simulink model "testing"  (R2023a)
settings: Solver=FixedStepAuto  StartTime=0.0  StopTime=5  FixedStep=0.00025  RelTol=1e-3
InitFcn:
  | addpath(fullfile(matlabroot,'toolbox/physmod/sm/sli/m'))
model workspace (MAT data in the model file):
  battery_cap = 500
  load = 500
libraries: fl_lib x73, ee_lib x11, nesl_utility x6, batteryecm_lib x2
settings Model: Creator=mluser  LastModifiedBy=mluser
settings OptimizationCC: ReuseModelBlockBuffer=off
settings SimscapeCC: SimscapeLogType=all  SimscapeLogLimitData=off

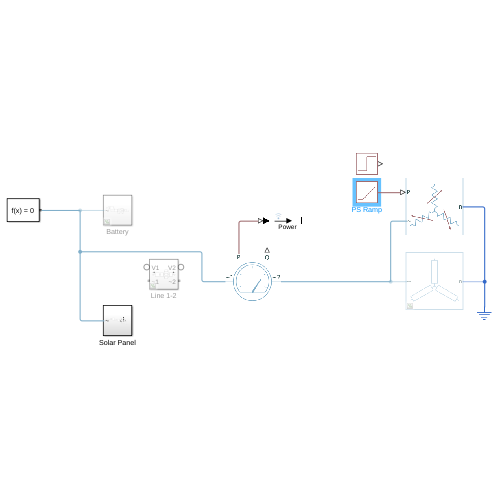
[thumbnail: Simulink's stored preview of the top-level diagram]
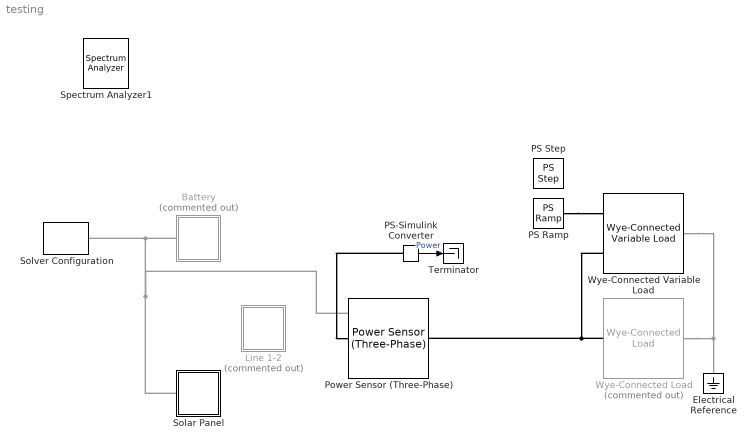
== system testing ==
  Battery : Subsystem  Commented=on
  Electrical Reference : fl_lib/Electrical/Electrical Elements/Electrical Reference
  Line 1-2 : Subsystem  Commented=on
  PS Ramp : fl_lib/Physical Signals/Sources/PS Ramp  slope=200 MW/s  start_time=0 s  initial_output=0 MW
  PS Step : fl_lib/Physical Signals/Sources/PS Step  step_time=1 s  initial_value=400 MW  final_value=1000 MW
  PS-Simulink Converter : nesl_utility/PS-Simulink Converter  PhysicalDomain=network_engine_domain  SubClassName=ps_output  LeftPortType=input  RightPortType=output  PseudoPeriodic=off  Frequencies=[]  VectorFormat=inherit  Unit=inherit  AffineConversion=off
  Power Sensor (Three-Phase) : ee_lib/Sensors & Transducers/Power Sensor (Three-Phase)  load_type=ee.enum.passive.type_balanced.balanced  f0=60 Hz  config=ee.enum.with_neutral.no  rho=1
      settings: InternalSimscapePortConfiguration="{\"Bottom\":[],\"Left\":[{\"id\":\"N1\",\"label\":\"~1\",\"type\":\"foundation.electrical.three_phase\"}],\"Right\":[{\"id\":\"N2\",\"label\":\"~2\",\"type\":\"foundation.electrical.three_phase\"}],\"Top\":[{\"id\":\"Pm\",\"label\":\"P\",\"type\":\"output\"},{\"id\":\"Qm\",\"label\":\"Q\",\"type\":\"output\"}]}"
  Solar Panel : Subsystem
  Solver Configuration : nesl_utility/Solver Configuration  PhysicalDomain=network_engine_domain  SubClassName=solver  LeftPortType=input  RightPortType=generic  Tones=[]  Harmonics=[]  SimulateNoise=off  Profile=off  UseLocalSampling=off  EnableSwitchedLinearOptims=on  FrequencyDomain=off  UseCCode=off  RelTol=0.001  AbsTol=0.001  MinStep=1e-09  ToWorkspace=off  RevertToSquareIcSolve=off  NumHomotopyIterations=100  PhasorMode=off  PhasorModeNumHarmonics=1  ConsistencySolver=NEWTON_XTOL_AFTER_FTOL  IndexReductionMethod=DerivativeReplacement  DoDC=off  ResidualTolerance=1e-09  ConsistencyTolSource=GLOBAL  ConsistencyAbsTol=0.001  ConsistencyRelTol=0.001  ConsistencyTolFactor=0.001  UseLocalSolver=off  LocalSolverChoice=NE_BACKWARD_EULER_ADVANCER  ResolveIndetEquations=on  FunctionEvalNumThread=1  LocalSolverSampleTime=0.001  DoFixedCost=off  MaxNonlinIter=3  MaxModeIter=2  ComputeImpulses=off  ImpulseIterations=2  LinearAlgebra=auto  LinearAlgebraNumThread=0  EquationFormulation=NE_TIME_EF  DelaysMemoryBudget=1024  AutomaticFiltering=on  FilteringTimeConstant=0.001  PartitionStorageMethod=AS_NEEDED  PartitionMemoryBudget=1024  PartitionMethod=ROBUST
  Terminator : Terminator
  Wye-Connected Variable Load : ee_lib/Passive/RLC Assemblies/Wye-Connected Variable Load  VRated=350*sqrt(3) kV  Pmin=1000 W
      settings: InternalSimscapePortConfiguration="{\"Bottom\":[],\"Left\":[{\"id\":\"P\",\"label\":\"P\",\"type\":\"input\"},{\"id\":\"N\",\"label\":\"~\",\"type\":\"foundation.electrical.three_phase\"}],\"Right\":[{\"id\":\"n\",\"label\":\"n\",\"type\":\"foundation.electrical.electrical\"}],\"Top\":[]}"
  Wye-Connected Load : ee_lib/Passive/RLC Assemblies/Wye-Connected Load  Commented=on  parameterization=ee.enum.rlc.parameterization.ratedpower  component_structure=ee.enum.rlc.structure.R  component_structure_PQ=ee.enum.rlc.structure.R  R=1 Ohm  L=1e-3 H  C=1e-6 F  VRated=350*sqrt(3) kV  FRated=60 Hz  P=load MW  Qpos=1e2 A*V  Qneg=-1e2 A*V  R_parasitic=0 Ohm  G_parasitic=0 1/Ohm  R_parasitic_PQ=0 Ohm  G_parasitic_PQ=0 1/Ohm  Vmag0=24e3 V  Vang0=0 deg  Freq0=60 Hz  IL_specify=off  IL_priority=High  IL=[0, 0, 0] A  IL_nominal_specify=off  IL_nominal_unit=A  IL_nominal_value=1  VC_specify=off  VC_priority=High  VC=[0, 0, 0] V  VC_nominal_specify=off  VC_nominal_unit=V  VC_nominal_value=1
  Spectrum Analyzer1 : SpectrumAnalyzer  IOType=viewer  WindowPosition=[692 368 558 418]  Method=Welch  AveragingMethod=Running
      settings: OpenAtSimulationStart=off
  wires:
  PS-Simulink Converter/1 -> Terminator/1  "Power"
  connections:
  Battery/LConn1 -- Power Sensor (Three-Phase)/LConn1 -- Solar Panel/LConn1 -- Solver Configuration/RConn1
  Wye-Connected Variable Load/LConn2 -- Power Sensor (Three-Phase)/RConn1 -- Wye-Connected Load/LConn1
  PS Ramp/RConn1 -- Wye-Connected Variable Load/LConn1
  Wye-Connected Load/RConn1 -- Electrical Reference/LConn1 -- Wye-Connected Variable Load/RConn1
  PS-Simulink Converter/LConn1 -- Power Sensor (Three-Phase)/LConn2

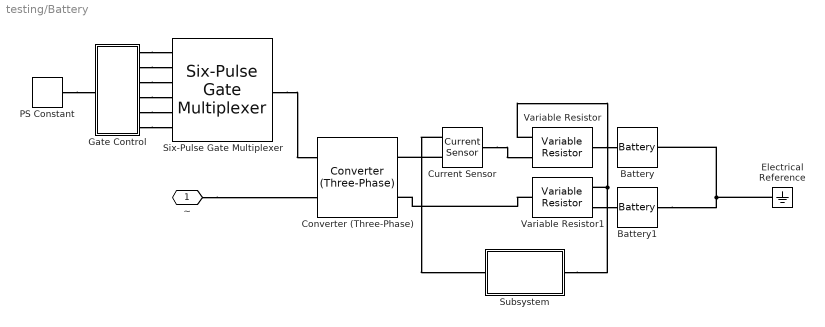
== system testing/Battery ==
  Battery : batteryecm_lib/Battery  Vnom=494.97 kV  prm_dir=simscape.enum.battery.prm_dir.disabled  R1_dis=2 Ohm  R1_ch=2 Ohm  R1=0.17 Ohm  prm_AH=simscape.enum.battery.prm_AH.infinite  AH=50 A*hr  V1=11.5 V  AH1=25 A*hr  prm_R2=simscape.enum.battery.prm_R2.disabled  R2=2000 Ohm  Tmeas=298.15 K  charge_measurement_port=simscape.enum.battery.enable.no  prm_dyn=simscape.enum.battery.prm_dyn.off  Rp1=0.005 Ohm  tau1=30 s  Rp2=0.005 Ohm  tau2=30 s  Rp3=0.005 Ohm  tau3=30 s  Rp4=0.005 Ohm  tau4=30 s  Rp5=0.005 Ohm  tau5=30 s  prm_fade=simscape.enum.battery.prm_fade.disabled  N_fade=100  AH_fade=45 A*hr  R1_fade=2.02 Ohm  R1_ch_fade=2.02 Ohm  V1_fade=10.35 V  prm_age=simscape.enum.battery.prm_age.disabled  prm_age_OCV=simscape.enum.battery.prm_age_OCV.OCV  OCV_age=0.9  SOC_age=60  Tmeas_age=298.15 K  delta_time_age_vec=[0] d  temperature_age_vec=[273] K  OCV_scaling_age=2.2134e6  OCV_offset_age=1.632e6  temp_exp_age=0.515833569 V  t_exp_age=0.75  Vnom_T2=12 V  R1_T2=2.2 Ohm  R1_T2_dis=2.2 Ohm  R1_T2_ch=2.2 Ohm  V1_T2=11.4 V  R2_T2=2200 Ohm  Rp1_T2=0.005 Ohm  tau1_T2=30 s  Rp2_T2=0.005 Ohm  tau2_T2=30 s  Rp3_T2=0.005 Ohm  tau3_T2=30 s  Rp4_T2=0.005 Ohm  tau4_T2=30 s  Rp5_T2=0.005 Ohm  tau5_T2=30 s  Tmeas2=273.15 K  thermal_port=simscape.enum.thermaleffects.omit  thermal_mass=30000 J/K  i_specify=off  i_priority=None  i=0 A  i_nominal_specify=off  i_nominal_unit=A  i_nominal_value=1  v_specify=off  v_priority=None  v=0 V  v_nominal_specify=off  v_nominal_unit=V  v_nominal_value=1  charge_specify=off  charge_priority=High  charge=50 A*hr  charge_nominal_specify=off  charge_nominal_unit=A*hr  charge_nominal_value=1  num_cycles_specify=off  num_cycles_priority=High  num_cycles=0  num_cycles_nominal_specify=off  num_cycles_nominal_unit=1  num_cycles_nominal_value=1  temperature_specify=off  temperature_priority=High  temperature=298.15 K  temperature_nominal_specify=off  temperature_nominal_unit=K  temperature_nominal_value=1
  Battery1 : batteryecm_lib/Battery  Vnom=494.97 kV  prm_dir=simscape.enum.battery.prm_dir.disabled  R1_dis=2 Ohm  R1_ch=2 Ohm  R1=0.17 Ohm  prm_AH=simscape.enum.battery.prm_AH.infinite  AH=50 A*hr  V1=11.5 V  AH1=25 A*hr  prm_R2=simscape.enum.battery.prm_R2.disabled  R2=2000 Ohm  Tmeas=298.15 K  charge_measurement_port=simscape.enum.battery.enable.no  prm_dyn=simscape.enum.battery.prm_dyn.off  Rp1=0.005 Ohm  tau1=30 s  Rp2=0.005 Ohm  tau2=30 s  Rp3=0.005 Ohm  tau3=30 s  Rp4=0.005 Ohm  tau4=30 s  Rp5=0.005 Ohm  tau5=30 s  prm_fade=simscape.enum.battery.prm_fade.disabled  N_fade=100  AH_fade=45 A*hr  R1_fade=2.02 Ohm  R1_ch_fade=2.02 Ohm  V1_fade=10.35 V  prm_age=simscape.enum.battery.prm_age.disabled  prm_age_OCV=simscape.enum.battery.prm_age_OCV.OCV  OCV_age=0.9  SOC_age=60  Tmeas_age=298.15 K  delta_time_age_vec=[0] d  temperature_age_vec=[273] K  OCV_scaling_age=2.2134e6  OCV_offset_age=1.632e6  temp_exp_age=0.515833569 V  t_exp_age=0.75  Vnom_T2=12 V  R1_T2=2.2 Ohm  R1_T2_dis=2.2 Ohm  R1_T2_ch=2.2 Ohm  V1_T2=11.4 V  R2_T2=2200 Ohm  Rp1_T2=0.005 Ohm  tau1_T2=30 s  Rp2_T2=0.005 Ohm  tau2_T2=30 s  Rp3_T2=0.005 Ohm  tau3_T2=30 s  Rp4_T2=0.005 Ohm  tau4_T2=30 s  Rp5_T2=0.005 Ohm  tau5_T2=30 s  Tmeas2=273.15 K  thermal_port=simscape.enum.thermaleffects.omit  thermal_mass=30000 J/K  i_specify=off  i_priority=None  i=0 A  i_nominal_specify=off  i_nominal_unit=A  i_nominal_value=1  v_specify=off  v_priority=None  v=0 V  v_nominal_specify=off  v_nominal_unit=V  v_nominal_value=1  charge_specify=off  charge_priority=High  charge=50 A*hr  charge_nominal_specify=off  charge_nominal_unit=A*hr  charge_nominal_value=1  num_cycles_specify=off  num_cycles_priority=High  num_cycles=0  num_cycles_nominal_specify=off  num_cycles_nominal_unit=1  num_cycles_nominal_value=1  temperature_specify=off  temperature_priority=High  temperature=298.15 K  temperature_nominal_specify=off  temperature_nominal_unit=K  temperature_nominal_value=1
  Converter (Three-Phase) : ee_lib/Semiconductors & Converters/Converters/Converter (Three-Phase)  port_option=ee.enum.threePhasePort.composite  device_type=ee.enum.converters.switchingdevice.averaged  K=0  Vf=0.8 V  Ron=1e-9 mOhm  Rds=0.001 Ohm  Goff=1e-6 1/Ohm  Vgt=1 V  Vgt_off=-1 V  Ih=1 A  Vth=6 V  diode_param=ee.enum.converters.protectiondiode.none  diode_Vf=1 MV  diode_Ron=0.001 Ohm  diode_Goff=1e-5 1/Ohm  diode_C=50 nF  diode_iRM=-235 A  diode_iF=300 A  diode_idot=-50 A/us  diode_trr_param=ee.enum.converters.diodetrr.trr_factor  diode_trr_factor=3  diode_trr=15 us  diode_Qrr=1500 s*uA  snubber_type=ee.enum.converters.snubber.exclude  Cs=1e-7 F  Rs=0.1 Ohm
  Current Sensor : fl_lib/Electrical/Electrical Sensors/Current Sensor
  Electrical Reference : fl_lib/Electrical/Electrical Elements/Electrical Reference
  Gate Control : Subsystem
  PS Constant : fl_lib/Physical Signals/Sources/PS Constant  constant=1
  Six-Pulse Gate Multiplexer : ee_lib/Semiconductors & Converters/Converters/Six-Pulse Gate Multiplexer  port_option=ee.enum.controlport.ps
  Subsystem : Subsystem
  Variable Resistor : fl_lib/Electrical/Electrical Elements/Variable Resistor  Rmin=0 Ohm  i_specify=off  i_priority=None  i=0 A  i_nominal_specify=off  i_nominal_unit=A  i_nominal_value=1  v_specify=off  v_priority=None  v=0 V  v_nominal_specify=off  v_nominal_unit=V  v_nominal_value=1
  Variable Resistor1 : fl_lib/Electrical/Electrical Elements/Variable Resistor  Rmin=0 Ohm  i_specify=off  i_priority=None  i=0 A  i_nominal_specify=off  i_nominal_unit=A  i_nominal_value=1  v_specify=off  v_priority=None  v=0 V  v_nominal_specify=off  v_nominal_unit=V  v_nominal_value=1
  ~ : PMIOPort  Side=Left
  connections:
  Six-Pulse Gate Multiplexer/RConn1 -- Converter (Three-Phase)/LConn1
  ~/RConn1 -- Converter (Three-Phase)/LConn2
  Gate Control/RConn1 -- Six-Pulse Gate Multiplexer/LConn1
  Gate Control/RConn2 -- Six-Pulse Gate Multiplexer/LConn2
  Gate Control/RConn3 -- Six-Pulse Gate Multiplexer/LConn3
  Gate Control/RConn4 -- Six-Pulse Gate Multiplexer/LConn4
  Gate Control/RConn5 -- Six-Pulse Gate Multiplexer/LConn5
  Gate Control/RConn6 -- Six-Pulse Gate Multiplexer/LConn6
  PS Constant/RConn1 -- Gate Control/LConn1
  Battery1/LConn1 -- Battery/RConn1 -- Electrical Reference/LConn1
  Current Sensor/RConn2 -- Converter (Three-Phase)/RConn1
  Variable Resistor/RConn1 -- Battery/LConn1
  Variable Resistor1/RConn1 -- Converter (Three-Phase)/RConn2
  Variable Resistor1/LConn2 -- Battery1/RConn1
  Current Sensor/LConn1 -- Variable Resistor/LConn2
  Current Sensor/RConn1 -- Subsystem/LConn1
  Subsystem/RConn1 -- Variable Resistor/LConn1 -- Variable Resistor1/LConn1

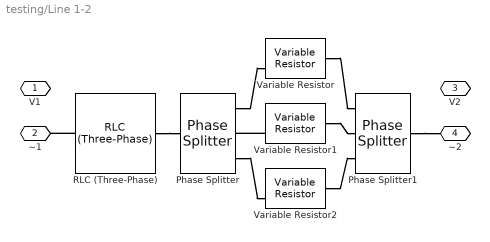
== system testing/Line 1-2 ==
  Phase Splitter : ee_lib/Connectors & References/Phase Splitter
  Phase Splitter1 : ee_lib/Connectors & References/Phase Splitter
  RLC (Three-Phase) : ee_lib/Passive/RLC Assemblies/RLC (Three-Phase)  component_structure=ee.enum.rlc.structure.SeriesRL  R=10 Ohm  L=5e-3 H  C=1e-6 F  R_parasitic=0 Ohm  G_parasitic=0 1/Ohm  IL_specify=off  IL_priority=High  IL=[0, 0, 0] A  IL_nominal_specify=off  IL_nominal_unit=A  IL_nominal_value=1  VC_specify=off  VC_priority=High  VC=[0, 0, 0] V  VC_nominal_specify=off  VC_nominal_unit=V  VC_nominal_value=1
      settings: InternalSimscapePortConfiguration="{\"Bottom\":[],\"Left\":[{\"id\":\"N1\",\"label\":\"~1\",\"type\":\"foundation.electrical.three_phase\"}],\"Right\":[{\"id\":\"N2\",\"label\":\"~2\",\"type\":\"foundation.electrical.three_phase\"}],\"Top\":[]}"
  Variable Resistor : fl_lib/Electrical/Electrical Elements/Variable Resistor  Rmin=0 Ohm  i_specify=off  i_priority=None  i=0 A  i_nominal_specify=off  i_nominal_unit=A  i_nominal_value=1  v_specify=off  v_priority=None  v=0 V  v_nominal_specify=off  v_nominal_unit=V  v_nominal_value=1
  Variable Resistor1 : fl_lib/Electrical/Electrical Elements/Variable Resistor  Rmin=0 Ohm  i_specify=off  i_priority=None  i=0 A  i_nominal_specify=off  i_nominal_unit=A  i_nominal_value=1  v_specify=off  v_priority=None  v=0 V  v_nominal_specify=off  v_nominal_unit=V  v_nominal_value=1
  Variable Resistor2 : fl_lib/Electrical/Electrical Elements/Variable Resistor  Rmin=0 Ohm  i_specify=off  i_priority=None  i=0 A  i_nominal_specify=off  i_nominal_unit=A  i_nominal_value=1  v_specify=off  v_priority=None  v=0 V  v_nominal_specify=off  v_nominal_unit=V  v_nominal_value=1
  V1 : PMIOPort  Side=Left
  ~1 : PMIOPort  Port=2  Side=Left
  V2 : PMIOPort  Port=3  Side=Right
  ~2 : PMIOPort  Port=4  Side=Right
  connections:
  RLC (Three-Phase)/RConn1 -- Phase Splitter/LConn1
  RLC (Three-Phase)/LConn1 -- ~1/RConn1
  Phase Splitter1/LConn1 -- ~2/RConn1
  Phase Splitter/RConn1 -- Variable Resistor/LConn2
  Variable Resistor/RConn1 -- Phase Splitter1/RConn1
  Variable Resistor1/LConn2 -- Phase Splitter/RConn2
  Variable Resistor1/RConn1 -- Phase Splitter1/RConn2
  Phase Splitter/RConn3 -- Variable Resistor2/LConn2
  Variable Resistor2/RConn1 -- Phase Splitter1/RConn3

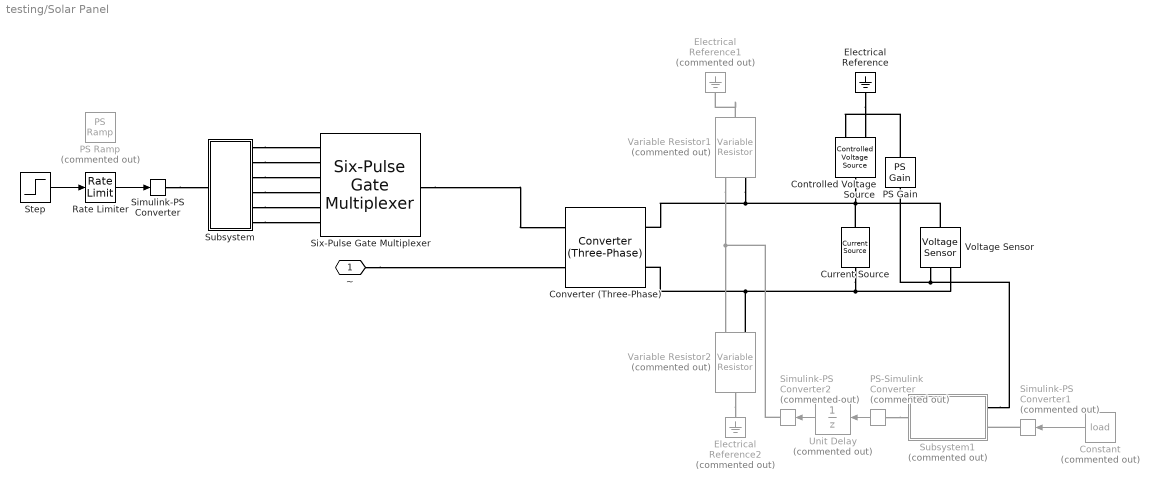
== system testing/Solar Panel ==
  Constant : Constant  Commented=on  Value=load  VectorParams1D=off
  Controlled Voltage Source : fl_lib/Electrical/Electrical Sources/Controlled Voltage Source
  Converter (Three-Phase) : ee_lib/Semiconductors & Converters/Converters/Converter (Three-Phase)  port_option=ee.enum.threePhasePort.composite  device_type=ee.enum.converters.switchingdevice.averaged  K=0  Vf=0.8 V  Ron=1e-9 Ohm  Rds=0.001 Ohm  Goff=1e-6 1/Ohm  Vgt=1 V  Vgt_off=-1 V  Ih=1 A  Vth=6 V  diode_param=ee.enum.converters.protectiondiode.none  diode_Vf=1 MV  diode_Ron=0.001 Ohm  diode_Goff=1e-5 1/Ohm  diode_C=50 nF  diode_iRM=-235 A  diode_iF=300 A  diode_idot=-50 A/us  diode_trr_param=ee.enum.converters.diodetrr.trr_factor  diode_trr_factor=3  diode_trr=15 us  diode_Qrr=1500 s*uA  snubber_type=ee.enum.converters.snubber.exclude  Cs=1e-7 F  Rs=0.1 Ohm
  Current Source : ee_lib/Sources/Current Source  dc_current=load/(2*350*sqrt(2)) kA  ac_current=0 A  ac_shift=0 rad  ac_frequency=60 Hz  noise_mode=ee.enum.sources.noise.Disabled  PSD=0 A^2/Hz  sample_time=1e-3 s  repeatability=ee.enum.sources.repeatability.NotRepeatable  user_seed=0  auto_seed=2715962282  i_specify=off  i_priority=None  i=0 A  i_nominal_specify=off  i_nominal_unit=A  i_nominal_value=1  v_specify=off  v_priority=None  v=0 V  v_nominal_specify=off  v_nominal_unit=V  v_nominal_value=1
  Electrical Reference : fl_lib/Electrical/Electrical Elements/Electrical Reference
  Electrical Reference1 : fl_lib/Electrical/Electrical Elements/Electrical Reference  Commented=on
  Electrical Reference2 : fl_lib/Electrical/Electrical Elements/Electrical Reference  Commented=on
  PS Gain : fl_lib/Physical Signals/Functions/PS Gain  gain=0.5
  PS Ramp : fl_lib/Physical Signals/Sources/PS Ramp  Commented=on  slope=0.1 1/s  start_time=1 s  initial_output=1
  PS-Simulink Converter : nesl_utility/PS-Simulink Converter  Commented=on  PhysicalDomain=network_engine_domain  SubClassName=ps_output  LeftPortType=input  RightPortType=output  PseudoPeriodic=off  Frequencies=[]  VectorFormat=inherit  Unit=inherit  AffineConversion=off
  Rate Limiter : RateLimiter  RisingSlewLimit=0.3  FallingSlewLimit=-0.3  SampleTimeMode=inherited
  Simulink-PS Converter : nesl_utility/Simulink-PS Converter  PhysicalDomain=network_engine_domain  SubClassName=ps_input  LeftPortType=input  RightPortType=output  PseudoPeriodic=off  Frequencies=[]  NoiseDistribution=none  NoiseParameters=[]  Unit=1  AffineConversion=off  FilteringAndDerivatives=provide  SimscapeFilterOrder=1  InputFilterTimeConstant=0.001  UdotUserProvided=0
  Simulink-PS Converter1 : nesl_utility/Simulink-PS Converter  Commented=on  PhysicalDomain=network_engine_domain  SubClassName=ps_input  LeftPortType=input  RightPortType=output  PseudoPeriodic=off  Frequencies=[]  NoiseDistribution=none  NoiseParameters=[]  Unit=MW  AffineConversion=off  FilteringAndDerivatives=provide  SimscapeFilterOrder=1  InputFilterTimeConstant=0.001  UdotUserProvided=0
  Simulink-PS Converter2 : nesl_utility/Simulink-PS Converter  Commented=on  PhysicalDomain=network_engine_domain  SubClassName=ps_input  LeftPortType=input  RightPortType=output  PseudoPeriodic=off  Frequencies=[]  NoiseDistribution=none  NoiseParameters=[]  Unit=Ohm  AffineConversion=off  FilteringAndDerivatives=provide  SimscapeFilterOrder=1  InputFilterTimeConstant=0.001  UdotUserProvided=0
  Six-Pulse Gate Multiplexer : ee_lib/Semiconductors & Converters/Converters/Six-Pulse Gate Multiplexer  port_option=ee.enum.controlport.ps
  Step : Step  Time=0  Before=1  SampleTime=0
  Subsystem : Subsystem
  Subsystem1 : Subsystem  Commented=on
  Unit Delay : UnitDelay  Commented=on  InitialCondition=1e9  SampleTime=-1  HasFrameUpgradeWarning=on
  Variable Resistor1 : fl_lib/Electrical/Electrical Elements/Variable Resistor  Commented=on  Rmin=0 Ohm  i_specify=off  i_priority=None  i=0 A  i_nominal_specify=off  i_nominal_unit=A  i_nominal_value=1  v_specify=off  v_priority=None  v=0 V  v_nominal_specify=off  v_nominal_unit=V  v_nominal_value=1
  Variable Resistor2 : fl_lib/Electrical/Electrical Elements/Variable Resistor  Commented=on  Rmin=0 Ohm  i_specify=off  i_priority=None  i=0 A  i_nominal_specify=off  i_nominal_unit=A  i_nominal_value=1  v_specify=off  v_priority=None  v=0 V  v_nominal_specify=off  v_nominal_unit=V  v_nominal_value=1
  Voltage Sensor : fl_lib/Electrical/Electrical Sensors/Voltage Sensor
  ~ : PMIOPort  Side=Left
  wires:
  Rate Limiter/1 -> Simulink-PS Converter/1
  Step/1 -> Rate Limiter/1
  Constant/1 -> Simulink-PS Converter1/1
  PS-Simulink Converter/1 -> Unit Delay/1
  Unit Delay/1 -> Simulink-PS Converter2/1
  connections:
  Voltage Sensor/RConn2 -- Current Source/RConn1 -- Variable Resistor2/LConn2 -- Converter (Three-Phase)/RConn2
  Voltage Sensor/LConn1 -- Current Source/LConn1 -- Converter (Three-Phase)/RConn1 -- Variable Resistor1/LConn2 -- Controlled Voltage Source/LConn1
  Voltage Sensor/RConn1 -- Subsystem1/LConn1 -- PS Gain/LConn1
  ~/RConn1 -- Converter (Three-Phase)/LConn2
  Six-Pulse Gate Multiplexer/RConn1 -- Converter (Three-Phase)/LConn1
  PS Gain/RConn1 -- Controlled Voltage Source/RConn1
  Electrical Reference/LConn1 -- Controlled Voltage Source/RConn2
  Subsystem/RConn1 -- Six-Pulse Gate Multiplexer/LConn1
  Subsystem/RConn2 -- Six-Pulse Gate Multiplexer/LConn2
  Subsystem/RConn3 -- Six-Pulse Gate Multiplexer/LConn3
  Subsystem/RConn4 -- Six-Pulse Gate Multiplexer/LConn4
  Subsystem/RConn5 -- Six-Pulse Gate Multiplexer/LConn5
  Subsystem/RConn6 -- Six-Pulse Gate Multiplexer/LConn6
  Simulink-PS Converter/RConn1 -- Subsystem/LConn1
  Variable Resistor1/RConn1 -- Electrical Reference1/LConn1
  Variable Resistor2/RConn1 -- Electrical Reference2/LConn1
  Simulink-PS Converter1/RConn1 -- Subsystem1/LConn2
  PS-Simulink Converter/LConn1 -- Subsystem1/RConn1
  Simulink-PS Converter2/RConn1 -- Variable Resistor2/LConn1 -- Variable Resistor1/LConn1

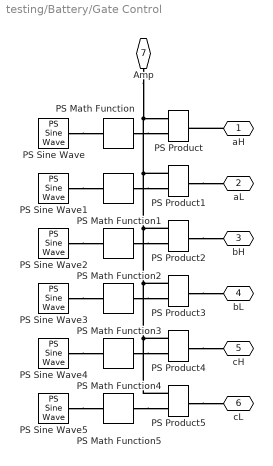
== system testing/Battery/Gate Control ==
  PS Math Function{,1..5} (6 alike) : fl_lib/Physical Signals/Functions/PS Math Function  fcn_choice=foundation.enum.math_function.square  v=1
  PS Product{,1..5} (6 alike) : fl_lib/Physical Signals/Functions/PS Product
  PS Sine Wave : fl_lib/Physical Signals/Sources/PS Sine Wave  amplitude=1  bias=0  frequency_spec=foundation.enum.frequencySpec.frequencySI  frequency_SI=30 Hz  frequency_angular=1 rad/s  phase=pi/2 rad
      settings: InternalSimscapePortConfiguration="{\"Bottom\":[],\"Left\":[],\"Right\":[{\"id\":\"O\",\"label\":\"\",\"type\":\"output\"}],\"Top\":[]}"
  PS Sine Wave1 : fl_lib/Physical Signals/Sources/PS Sine Wave  amplitude=1  bias=0  frequency_spec=foundation.enum.frequencySpec.frequencySI  frequency_SI=30 Hz  frequency_angular=1 rad/s  phase=0 rad
      settings: InternalSimscapePortConfiguration="{\"Bottom\":[],\"Left\":[],\"Right\":[{\"id\":\"O\",\"label\":\"\",\"type\":\"output\"}],\"Top\":[]}"
  PS Sine Wave2 : fl_lib/Physical Signals/Sources/PS Sine Wave  amplitude=1  bias=0  frequency_spec=foundation.enum.frequencySpec.frequencySI  frequency_SI=30 Hz  frequency_angular=1 rad/s  phase=2*pi/3+pi/2 rad
      settings: InternalSimscapePortConfiguration="{\"Bottom\":[],\"Left\":[],\"Right\":[{\"id\":\"O\",\"label\":\"\",\"type\":\"output\"}],\"Top\":[]}"
  PS Sine Wave3 : fl_lib/Physical Signals/Sources/PS Sine Wave  amplitude=1  bias=0  frequency_spec=foundation.enum.frequencySpec.frequencySI  frequency_SI=30 Hz  frequency_angular=1 rad/s  phase=2*pi/3 rad
      settings: InternalSimscapePortConfiguration="{\"Bottom\":[],\"Left\":[],\"Right\":[{\"id\":\"O\",\"label\":\"\",\"type\":\"output\"}],\"Top\":[]}"
  PS Sine Wave4 : fl_lib/Physical Signals/Sources/PS Sine Wave  amplitude=1  bias=0  frequency_spec=foundation.enum.frequencySpec.frequencySI  frequency_SI=30 Hz  frequency_angular=1 rad/s  phase=-2*pi/3+pi/2 rad
      settings: InternalSimscapePortConfiguration="{\"Bottom\":[],\"Left\":[],\"Right\":[{\"id\":\"O\",\"label\":\"\",\"type\":\"output\"}],\"Top\":[]}"
  PS Sine Wave5 : fl_lib/Physical Signals/Sources/PS Sine Wave  amplitude=1  bias=0  frequency_spec=foundation.enum.frequencySpec.frequencySI  frequency_SI=30 Hz  frequency_angular=1 rad/s  phase=-2*pi/3 rad
      settings: InternalSimscapePortConfiguration="{\"Bottom\":[],\"Left\":[],\"Right\":[{\"id\":\"O\",\"label\":\"\",\"type\":\"output\"}],\"Top\":[]}"
  aH : PMIOPort  Side=Right
  aL : PMIOPort  Port=2  Side=Right
  bH : PMIOPort  Port=3  Side=Right
  bL : PMIOPort  Port=4  Side=Right
  cH : PMIOPort  Port=5  Side=Right
  cL : PMIOPort  Port=6  Side=Right
  Amp : PMIOPort  Port=7  Side=Left
  connections:
  aH/RConn1 -- PS Product/RConn1
  PS Math Function/RConn1 -- PS Product/LConn2
  Amp/RConn1 -- PS Product/LConn1 -- PS Product1/LConn1 -- PS Product2/LConn1 -- PS Product3/LConn1 -- PS Product5/LConn1 -- PS Product4/LConn1
  PS Sine Wave/RConn1 -- PS Math Function/LConn1
  PS Math Function1/RConn1 -- PS Product1/LConn2
  PS Sine Wave1/RConn1 -- PS Math Function1/LConn1
  PS Product1/RConn1 -- aL/RConn1
  PS Math Function2/RConn1 -- PS Product2/LConn2
  PS Sine Wave2/RConn1 -- PS Math Function2/LConn1
  PS Product2/RConn1 -- bH/RConn1
  PS Math Function3/RConn1 -- PS Product3/LConn2
  PS Sine Wave3/RConn1 -- PS Math Function3/LConn1
  PS Product3/RConn1 -- bL/RConn1
  PS Math Function4/RConn1 -- PS Product4/LConn2
  PS Sine Wave4/RConn1 -- PS Math Function4/LConn1
  PS Math Function5/RConn1 -- PS Product5/LConn2
  PS Sine Wave5/RConn1 -- PS Math Function5/LConn1
  PS Product4/RConn1 -- cH/RConn1
  PS Product5/RConn1 -- cL/RConn1

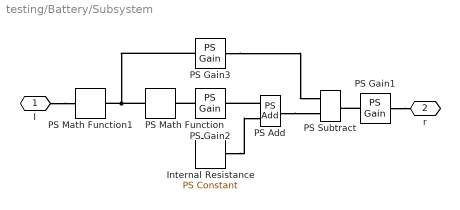
== system testing/Battery/Subsystem ==
  Internal Resistance : fl_lib/Physical Signals/Sources/PS Constant  constant=0.34 Ohm
  PS Add : fl_lib/Physical Signals/Functions/PS Add
  PS Gain1 : fl_lib/Physical Signals/Functions/PS Gain  gain=0.5
  PS Gain2 : fl_lib/Physical Signals/Functions/PS Gain  gain=battery_cap MW
  PS Gain3 : fl_lib/Physical Signals/Functions/PS Gain  gain=2*350*sqrt(2) kV
  PS Math Function : fl_lib/Physical Signals/Functions/PS Math Function  fcn_choice=foundation.enum.math_function.square  v=1
  PS Math Function1 : fl_lib/Physical Signals/Functions/PS Math Function  fcn_choice=foundation.enum.math_function.reciprocal  v=1
  PS Subtract : fl_lib/Physical Signals/Functions/PS Subtract
  I : PMIOPort  Side=Left
  r : PMIOPort  Port=2  Side=Right
  connections:
  I/RConn1 -- PS Math Function1/LConn1
  PS Gain1/LConn1 -- PS Subtract/RConn1
  PS Gain1/RConn1 -- r/RConn1
  PS Add/RConn1 -- PS Subtract/LConn2
  Internal Resistance/RConn1 -- PS Add/LConn2
  PS Math Function/LConn1 -- PS Gain3/LConn1 -- PS Math Function1/RConn1
  PS Gain2/LConn1 -- PS Math Function/RConn1
  PS Add/LConn1 -- PS Gain2/RConn1
  PS Gain3/RConn1 -- PS Subtract/LConn1

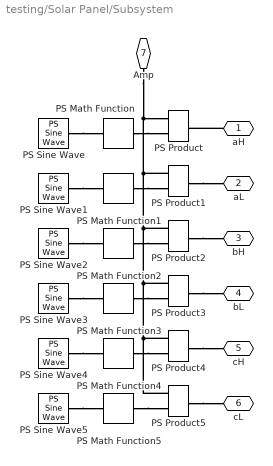
== system testing/Solar Panel/Subsystem ==
  PS Math Function{,1..5} (6 alike) : fl_lib/Physical Signals/Functions/PS Math Function  fcn_choice=foundation.enum.math_function.square  v=1
  PS Product{,1..5} (6 alike) : fl_lib/Physical Signals/Functions/PS Product
  PS Sine Wave : fl_lib/Physical Signals/Sources/PS Sine Wave  amplitude=1  bias=0  frequency_spec=foundation.enum.frequencySpec.frequencySI  frequency_SI=30 Hz  frequency_angular=1 rad/s  phase=pi/2 rad
      settings: InternalSimscapePortConfiguration="{\"Bottom\":[],\"Left\":[],\"Right\":[{\"id\":\"O\",\"label\":\"\",\"type\":\"output\"}],\"Top\":[]}"
  PS Sine Wave1 : fl_lib/Physical Signals/Sources/PS Sine Wave  amplitude=1  bias=0  frequency_spec=foundation.enum.frequencySpec.frequencySI  frequency_SI=30 Hz  frequency_angular=1 rad/s  phase=0 rad
      settings: InternalSimscapePortConfiguration="{\"Bottom\":[],\"Left\":[],\"Right\":[{\"id\":\"O\",\"label\":\"\",\"type\":\"output\"}],\"Top\":[]}"
  PS Sine Wave2 : fl_lib/Physical Signals/Sources/PS Sine Wave  amplitude=1  bias=0  frequency_spec=foundation.enum.frequencySpec.frequencySI  frequency_SI=30 Hz  frequency_angular=1 rad/s  phase=-2*pi/3+pi/2 rad
      settings: InternalSimscapePortConfiguration="{\"Bottom\":[],\"Left\":[],\"Right\":[{\"id\":\"O\",\"label\":\"\",\"type\":\"output\"}],\"Top\":[]}"
  PS Sine Wave3 : fl_lib/Physical Signals/Sources/PS Sine Wave  amplitude=1  bias=0  frequency_spec=foundation.enum.frequencySpec.frequencySI  frequency_SI=30 Hz  frequency_angular=1 rad/s  phase=-2*pi/3 rad
      settings: InternalSimscapePortConfiguration="{\"Bottom\":[],\"Left\":[],\"Right\":[{\"id\":\"O\",\"label\":\"\",\"type\":\"output\"}],\"Top\":[]}"
  PS Sine Wave4 : fl_lib/Physical Signals/Sources/PS Sine Wave  amplitude=1  bias=0  frequency_spec=foundation.enum.frequencySpec.frequencySI  frequency_SI=30 Hz  frequency_angular=1 rad/s  phase=2*pi/3+pi/2 rad
      settings: InternalSimscapePortConfiguration="{\"Bottom\":[],\"Left\":[],\"Right\":[{\"id\":\"O\",\"label\":\"\",\"type\":\"output\"}],\"Top\":[]}"
  PS Sine Wave5 : fl_lib/Physical Signals/Sources/PS Sine Wave  amplitude=1  bias=0  frequency_spec=foundation.enum.frequencySpec.frequencySI  frequency_SI=30 Hz  frequency_angular=1 rad/s  phase=2*pi/3 rad
      settings: InternalSimscapePortConfiguration="{\"Bottom\":[],\"Left\":[],\"Right\":[{\"id\":\"O\",\"label\":\"\",\"type\":\"output\"}],\"Top\":[]}"
  aH : PMIOPort  Side=Right
  aL : PMIOPort  Port=2  Side=Right
  bH : PMIOPort  Port=3  Side=Right
  bL : PMIOPort  Port=4  Side=Right
  cH : PMIOPort  Port=5  Side=Right
  cL : PMIOPort  Port=6  Side=Right
  Amp : PMIOPort  Port=7  Side=Left
  connections:
  aH/RConn1 -- PS Product/RConn1
  PS Math Function/RConn1 -- PS Product/LConn2
  Amp/RConn1 -- PS Product/LConn1 -- PS Product1/LConn1 -- PS Product2/LConn1 -- PS Product3/LConn1 -- PS Product5/LConn1 -- PS Product4/LConn1
  PS Sine Wave/RConn1 -- PS Math Function/LConn1
  PS Math Function1/RConn1 -- PS Product1/LConn2
  PS Sine Wave1/RConn1 -- PS Math Function1/LConn1
  PS Product1/RConn1 -- aL/RConn1
  PS Math Function2/RConn1 -- PS Product2/LConn2
  PS Sine Wave2/RConn1 -- PS Math Function2/LConn1
  PS Product2/RConn1 -- bH/RConn1
  PS Math Function3/RConn1 -- PS Product3/LConn2
  PS Sine Wave3/RConn1 -- PS Math Function3/LConn1
  PS Product3/RConn1 -- bL/RConn1
  PS Math Function4/RConn1 -- PS Product4/LConn2
  PS Sine Wave4/RConn1 -- PS Math Function4/LConn1
  PS Math Function5/RConn1 -- PS Product5/LConn2
  PS Sine Wave5/RConn1 -- PS Math Function5/LConn1
  PS Product4/RConn1 -- cH/RConn1
  PS Product5/RConn1 -- cL/RConn1

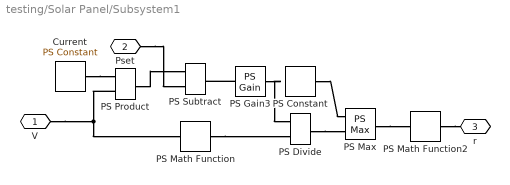
== system testing/Solar Panel/Subsystem1 ==
  Current : fl_lib/Physical Signals/Sources/PS Constant  constant=load/(2*350*sqrt(2)) kA
  PS Constant : fl_lib/Physical Signals/Sources/PS Constant  constant=1e-9 1/Ohm
  PS Divide : fl_lib/Physical Signals/Functions/PS Divide
  PS Gain3 : fl_lib/Physical Signals/Functions/PS Gain  gain=2
  PS Math Function : fl_lib/Physical Signals/Functions/PS Math Function  fcn_choice=foundation.enum.math_function.square  v=1
  PS Math Function2 : fl_lib/Physical Signals/Functions/PS Math Function  fcn_choice=foundation.enum.math_function.reciprocal  v=1
  PS Max : fl_lib/Physical Signals/Nonlinear Operators/PS Max
      settings: InternalSimscapePortConfiguration="{\"Bottom\":[],\"Left\":[{\"id\":\"I1\",\"label\":\"\",\"type\":\"input\"},{\"id\":\"I2\",\"label\":\"\",\"type\":\"input\"}],\"Right\":[{\"id\":\"O\",\"label\":\"\",\"type\":\"output\"}],\"Top\":[]}"
  PS Product : fl_lib/Physical Signals/Functions/PS Product
  PS Subtract : fl_lib/Physical Signals/Functions/PS Subtract
  V : PMIOPort  Side=Left
  Pset : PMIOPort  Port=2  Side=Left
  r : PMIOPort  Port=3  Side=Right
  connections:
  PS Math Function2/RConn1 -- r/RConn1
  V/RConn1 -- PS Product/LConn2 -- PS Math Function/LConn1
  PS Gain3/LConn1 -- PS Subtract/RConn1
  Current/RConn1 -- PS Product/LConn1
  PS Gain3/RConn1 -- PS Divide/LConn1
  PS Math Function/RConn1 -- PS Divide/LConn2
  Pset/RConn1 -- PS Subtract/LConn2
  PS Product/RConn1 -- PS Subtract/LConn1
  PS Max/RConn1 -- PS Math Function2/LConn1
  PS Divide/RConn1 -- PS Max/LConn2
  PS Constant/RConn1 -- PS Max/LConn1
